simulink library "Chip_Library"  (R2018b)
settings: Solver=VariableStepAuto  StartTime=0.0  StopTime=10.0  RelTol=1e-3
settings Model: Creator=jon  LastModifiedBy=jon
settings DebuggingCC: LibraryContextMissingDiagnostic=none
settings SFSimCC: SimUseLocalCustomCode=off
settings RTWCC: RTWUseLocalCustomCode=off

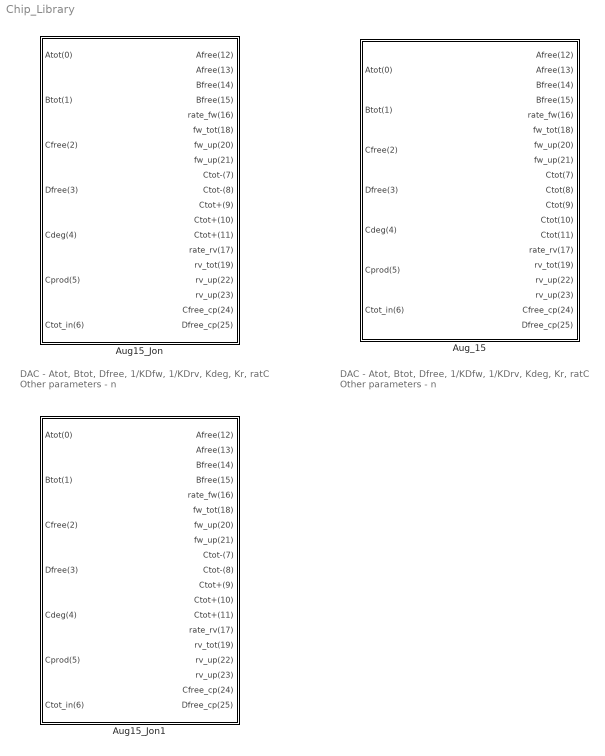
== system Chip_Library ==
  note: DAC - Atot, Btot, Dfree, 1/KDfw, 1/KDrv, Kdeg, Kr, ratC
      | Other parameters - n
  note: DAC - Atot, Btot, Dfree, 1/KDfw, 1/KDrv, Kdeg, Kr, ratC
      | Other parameters - n
  Aug15_Jon : Subsystem  mask{KDfw=1, KDrv=1, kr=1, kdeg=1, ratC=1, n=1, c_ic=0.01, A_FB_EN=0, B_FB_EN=0, FF_EN1=0, FF_EN2=0, FF_EN3=0, FF_EN4=0, Ctot_sw=0}
      mask prompts: KDfw "KD of forward reaction (KDfw)"; KDrv "KD of reverse reaction* (KDrv)"; kr "Reverse reaction rate (kr)"; kdeg "Degradation rate overall (kdeg)"; ratC "Degradation rate of C (ratC)"; n "Hill coefficient (n)"; c_ic "Initial condition of C (c_ic)"; A_FB_EN "Switch for Afree = Atot - ||| Ctot ||| (A_FB_EN)"; B_FB_EN "Switch for Bfree = Btot - ||| Ctot |||  (B_FB_EN)"; FF_EN1 "Switch for fw_up = C_prod - ||| rate_fw ||| (FF_EN1)"; FF_EN2 "Switch for fw_tot = C_prod + ||| rate_fw ||| (FF_EN2)"; FF_EN3 "Switch for rv_tot = C_deg+deg + ||| rate_rv ||| (FF_EN3)"; FF_EN4 "Switch for rv_up = C_deg+deg - ||| rate_rv ||| (FF_EN4)"; Ctot_sw "Switch for Ctot_in"
  Aug15_Jon1 : Subsystem  mask{Atot_cnst=0, Btot_cnst=0, Dfree_cnst=0, KDfw=1, KDrv=1, kr=1, kdeg=1, ratC=1, n=1, c_ic=0.01, A_FB_EN=0, B_FB_EN=0, sel_rate=1, sel_Ctot=1}
      mask prompts: Atot_cnst "Atot constant"; Btot_cnst "Btot constant"; Dfree_cnst "Dfree constant"; KDfw "KD of forward reaction (KDfw)"; KDrv "KD of reverse reaction* (KDrv)"; kr "Reverse reaction rate (kr)"; kdeg "Degradation rate overall (kdeg)"; ratC "Degradation rate of C (ratC)"; n "Hill coefficient (n)"; c_ic "Initial condition of C (c_ic)"; A_FB_EN "Switch for Afree = Atot - ||| Ctot ||| (A_FB_EN)"; B_FB_EN "Switch for Bfree = Btot - ||| Ctot |||  (B_FB_EN)"; sel_rate "fw_up, fw_tot, rv_tot, rv_up (Default=1: off on on off)"; sel_Ctot "Switch for Ctot_in (Default=1 : off)"
  Aug_15 : Subsystem  mask{KDfw=1, kr=1, kdeg=1, ratC=1, KDrv=1, n=1}

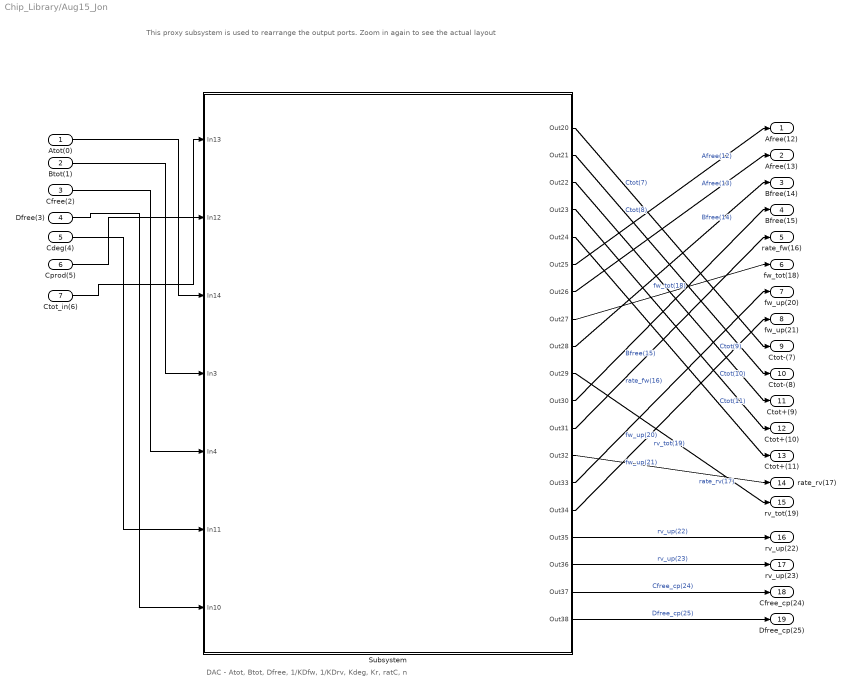
== system Chip_Library/Aug15_Jon ==
  note: This proxy subsystem is used to rearrange the output ports.
      | Zoom in again to see the actual layout
  note: DAC - Atot, Btot, Dfree, 1/KDfw, 1/KDrv, Kdeg, Kr, ratC, n
  Atot(0) : Inport
  Btot(1) : Inport  Port=2
  Cfree(2) : Inport  Port=3
  Dfree(3) : Inport  Port=4
  Cdeg(4) : Inport  Port=5
  Cprod(5) : Inport  Port=6
  Ctot_in(6) : Inport  Port=7
  Subsystem : Subsystem
  Afree(12) : Outport
  Afree(13) : Outport  Port=2
  Bfree(14) : Outport  Port=3
  Bfree(15) : Outport  Port=4
  rate_fw(16) : Outport  Port=5
  fw_tot(18) : Outport  Port=6
  fw_up(20) : Outport  Port=7
  fw_up(21) : Outport  Port=8
  Ctot-(7) : Outport  Port=9
  Ctot-(8) : Outport  Port=10
  Ctot+(9) : Outport  Port=11
  Ctot+(10) : Outport  Port=12
  Ctot+(11) : Outport  Port=13
  rate_rv(17) : Outport  Port=14
  rv_tot(19) : Outport  Port=15
  rv_up(22) : Outport  Port=16
  rv_up(23) : Outport  Port=17
  Cfree_cp(24) : Outport  Port=18
  Dfree_cp(25) : Outport  Port=19
  wires:
  Subsystem/8(Out27) -> fw_tot(18)/1  "fw_tot(18)"
  Subsystem/16(Out35) -> rv_up(22)/1  "rv_up(22)"
  Subsystem/3(Out22) -> Ctot+(9)/1  "Ctot(9)"
  Ctot_in(6)/1 -> Subsystem/1(In13)
  Cdeg(4)/1 -> Subsystem/6(In11)
  Cfree(2)/1 -> Subsystem/5(In4)
  Subsystem/9(Out28) -> Bfree(14)/1  "Bfree(14)"
  Atot(0)/1 -> Subsystem/3(In14)
  Subsystem/1(Out20) -> Ctot-(7)/1  "Ctot(7)"
  Btot(1)/1 -> Subsystem/4(In3)
  Subsystem/2(Out21) -> Ctot-(8)/1  "Ctot(8)"
  Subsystem/11(Out30) -> Bfree(15)/1  "Bfree(15)"
  Subsystem/18(Out37) -> Cfree_cp(24)/1  "Cfree_cp(24)"
  Subsystem/5(Out24) -> Ctot+(11)/1  "Ctot(11)"
  Dfree(3)/1 -> Subsystem/7(In10)
  Cprod(5)/1 -> Subsystem/2(In12)
  Subsystem/15(Out34) -> fw_up(21)/1  "fw_up(21)"
  Subsystem/4(Out23) -> Ctot+(10)/1  "Ctot(10)"
  Subsystem/19(Out38) -> Dfree_cp(25)/1  "Dfree_cp(25)"
  Subsystem/14(Out33) -> fw_up(20)/1  "fw_up(20)"
  Subsystem/6(Out25) -> Afree(12)/1  "Afree(12)"
  Subsystem/12(Out31) -> rate_fw(16)/1  "rate_fw(16)"
  Subsystem/7(Out26) -> Afree(13)/1  "Afree(13)"
  Subsystem/13(Out32) -> rate_rv(17)/1  "rate_rv(17)"
  Subsystem/17(Out36) -> rv_up(23)/1  "rv_up(23)"
  Subsystem/10(Out29) -> rv_tot(19)/1  "rv_tot(19)"

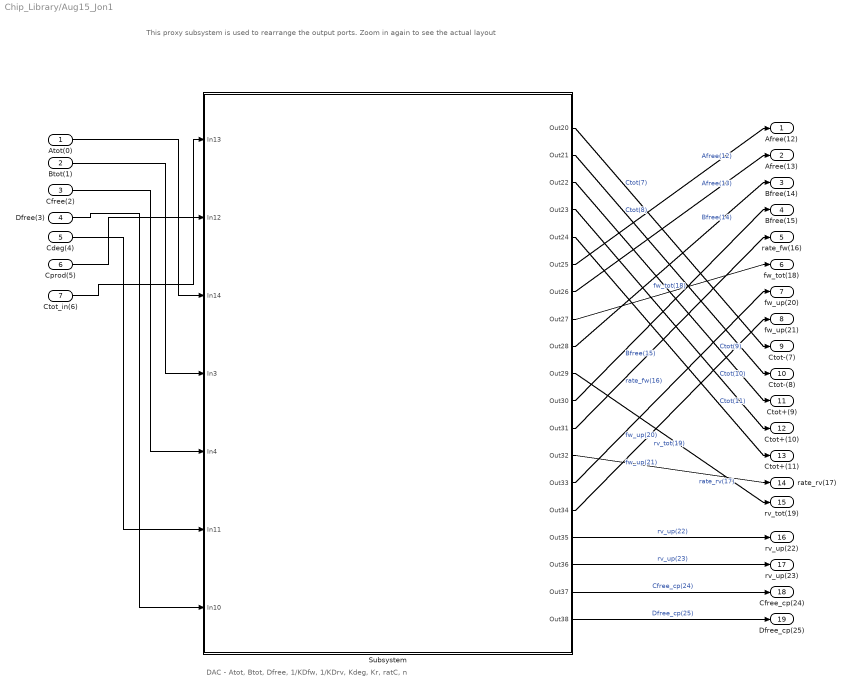
== system Chip_Library/Aug15_Jon1 ==
  note: This proxy subsystem is used to rearrange the output ports.
      | Zoom in again to see the actual layout
  note: DAC - Atot, Btot, Dfree, 1/KDfw, 1/KDrv, Kdeg, Kr, ratC, n
  Atot(0) : Inport
  Btot(1) : Inport  Port=2
  Cfree(2) : Inport  Port=3
  Dfree(3) : Inport  Port=4
  Cdeg(4) : Inport  Port=5
  Cprod(5) : Inport  Port=6
  Ctot_in(6) : Inport  Port=7
  Subsystem : Subsystem
  Afree(12) : Outport
  Afree(13) : Outport  Port=2
  Bfree(14) : Outport  Port=3
  Bfree(15) : Outport  Port=4
  rate_fw(16) : Outport  Port=5
  fw_tot(18) : Outport  Port=6
  fw_up(20) : Outport  Port=7
  fw_up(21) : Outport  Port=8
  Ctot-(7) : Outport  Port=9
  Ctot-(8) : Outport  Port=10
  Ctot+(9) : Outport  Port=11
  Ctot+(10) : Outport  Port=12
  Ctot+(11) : Outport  Port=13
  rate_rv(17) : Outport  Port=14
  rv_tot(19) : Outport  Port=15
  rv_up(22) : Outport  Port=16
  rv_up(23) : Outport  Port=17
  Cfree_cp(24) : Outport  Port=18
  Dfree_cp(25) : Outport  Port=19
  wires:
  Subsystem/8(Out27) -> fw_tot(18)/1  "fw_tot(18)"
  Subsystem/16(Out35) -> rv_up(22)/1  "rv_up(22)"
  Subsystem/3(Out22) -> Ctot+(9)/1  "Ctot(9)"
  Ctot_in(6)/1 -> Subsystem/1(In13)
  Cdeg(4)/1 -> Subsystem/6(In11)
  Cfree(2)/1 -> Subsystem/5(In4)
  Subsystem/9(Out28) -> Bfree(14)/1  "Bfree(14)"
  Atot(0)/1 -> Subsystem/3(In14)
  Subsystem/1(Out20) -> Ctot-(7)/1  "Ctot(7)"
  Btot(1)/1 -> Subsystem/4(In3)
  Subsystem/2(Out21) -> Ctot-(8)/1  "Ctot(8)"
  Subsystem/11(Out30) -> Bfree(15)/1  "Bfree(15)"
  Subsystem/18(Out37) -> Cfree_cp(24)/1  "Cfree_cp(24)"
  Subsystem/5(Out24) -> Ctot+(11)/1  "Ctot(11)"
  Dfree(3)/1 -> Subsystem/7(In10)
  Cprod(5)/1 -> Subsystem/2(In12)
  Subsystem/15(Out34) -> fw_up(21)/1  "fw_up(21)"
  Subsystem/4(Out23) -> Ctot+(10)/1  "Ctot(10)"
  Subsystem/19(Out38) -> Dfree_cp(25)/1  "Dfree_cp(25)"
  Subsystem/14(Out33) -> fw_up(20)/1  "fw_up(20)"
  Subsystem/6(Out25) -> Afree(12)/1  "Afree(12)"
  Subsystem/12(Out31) -> rate_fw(16)/1  "rate_fw(16)"
  Subsystem/7(Out26) -> Afree(13)/1  "Afree(13)"
  Subsystem/13(Out32) -> rate_rv(17)/1  "rate_rv(17)"
  Subsystem/17(Out36) -> rv_up(23)/1  "rv_up(23)"
  Subsystem/10(Out29) -> rv_tot(19)/1  "rv_tot(19)"

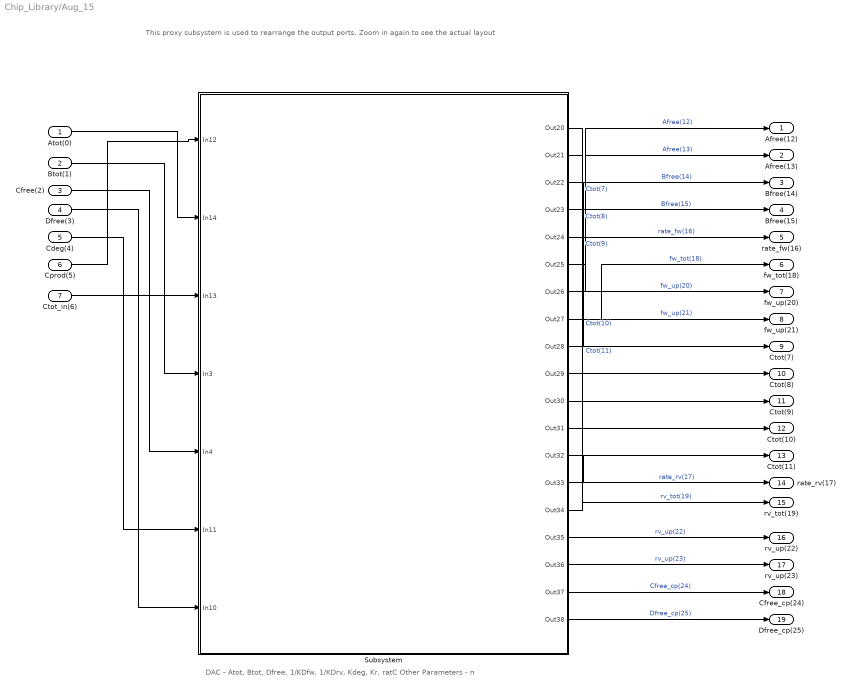
== system Chip_Library/Aug_15 ==
  note: This proxy subsystem is used to rearrange the output ports.
      | Zoom in again to see the actual layout
  note: DAC - Atot, Btot, Dfree, 1/KDfw, 1/KDrv, Kdeg, Kr, ratC
      | Other Parameters - n
  Atot(0) : Inport
  Btot(1) : Inport  Port=2
  Cfree(2) : Inport  Port=3
  Dfree(3) : Inport  Port=4
  Cdeg(4) : Inport  Port=5
  Cprod(5) : Inport  Port=6
  Ctot_in(6) : Inport  Port=7
  Subsystem : Subsystem
  Afree(12) : Outport
  Afree(13) : Outport  Port=2
  Bfree(14) : Outport  Port=3
  Bfree(15) : Outport  Port=4
  rate_fw(16) : Outport  Port=5
  fw_tot(18) : Outport  Port=6
  fw_up(20) : Outport  Port=7
  fw_up(21) : Outport  Port=8
  Ctot(7) : Outport  Port=9
  Ctot(8) : Outport  Port=10
  Ctot(9) : Outport  Port=11
  Ctot(10) : Outport  Port=12
  Ctot(11) : Outport  Port=13
  rate_rv(17) : Outport  Port=14
  rv_tot(19) : Outport  Port=15
  rv_up(22) : Outport  Port=16
  rv_up(23) : Outport  Port=17
  Cfree_cp(24) : Outport  Port=18
  Dfree_cp(25) : Outport  Port=19
  wires:
  Subsystem/8(Out27) -> fw_tot(18)/1  "fw_tot(18)"
  Subsystem/16(Out35) -> rv_up(22)/1  "rv_up(22)"
  Subsystem/3(Out22) -> Ctot(9)/1  "Ctot(9)"
  Ctot_in(6)/1 -> Subsystem/3(In13)
  Cdeg(4)/1 -> Subsystem/6(In11)
  Cfree(2)/1 -> Subsystem/5(In4)
  Subsystem/9(Out28) -> Bfree(14)/1  "Bfree(14)"
  Atot(0)/1 -> Subsystem/2(In14)
  Subsystem/1(Out20) -> Ctot(7)/1  "Ctot(7)"
  Btot(1)/1 -> Subsystem/4(In3)
  Subsystem/2(Out21) -> Ctot(8)/1  "Ctot(8)"
  Subsystem/11(Out30) -> Bfree(15)/1  "Bfree(15)"
  Subsystem/18(Out37) -> Cfree_cp(24)/1  "Cfree_cp(24)"
  Subsystem/5(Out24) -> Ctot(11)/1  "Ctot(11)"
  Dfree(3)/1 -> Subsystem/7(In10)
  Cprod(5)/1 -> Subsystem/1(In12)
  Subsystem/15(Out34) -> fw_up(21)/1  "fw_up(21)"
  Subsystem/4(Out23) -> Ctot(10)/1  "Ctot(10)"
  Subsystem/19(Out38) -> Dfree_cp(25)/1  "Dfree_cp(25)"
  Subsystem/14(Out33) -> fw_up(20)/1  "fw_up(20)"
  Subsystem/6(Out25) -> Afree(12)/1  "Afree(12)"
  Subsystem/12(Out31) -> rate_fw(16)/1  "rate_fw(16)"
  Subsystem/7(Out26) -> Afree(13)/1  "Afree(13)"
  Subsystem/13(Out32) -> rate_rv(17)/1  "rate_rv(17)"
  Subsystem/17(Out36) -> rv_up(23)/1  "rv_up(23)"
  Subsystem/10(Out29) -> rv_tot(19)/1  "rv_tot(19)"

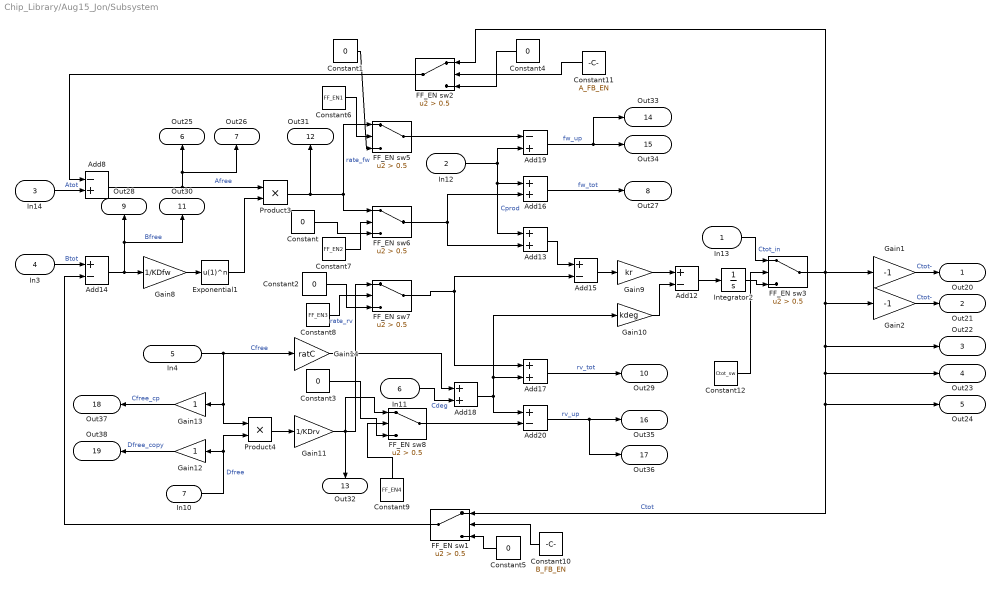
== system Chip_Library/Aug15_Jon/Subsystem ==
  In13 : Inport
  In12 : Inport  Port=2
  In14 : Inport  Port=3
  In3 : Inport  Port=4
  In4 : Inport  Port=5
  In11 : Inport  Port=6
  In10 : Inport  Port=7
  Add{12,14..15,20} (4 alike) : Sum  Inputs=+-
  Add{13,16..18} (4 alike) : Sum
  Add19 : Sum  Inputs=-+
  Add8 : Sum  Inputs=-+
  Constant{,1..5} (6 alike) : Constant  Value=0
  Constant10 : Constant  Value=B_FB_EN
  Constant11 : Constant  Value=A_FB_EN
  Constant12 : Constant  Value=Ctot_sw
  Constant6 : Constant  Value=FF_EN1
  Constant7 : Constant  Value=FF_EN2
  Constant8 : Constant  Value=FF_EN3
  Constant9 : Constant  Value=FF_EN4
  Exponential1 : Fcn  Expr=u(1)^n
  FF_EN sw{1..3,5..8} (7 alike) : Switch  Criteria=u2 > Threshold  Threshold=0.5
  Gain1 : Gain  Gain=-1
  Gain10 : Gain  Gain=kdeg
  Gain11 : Gain  Gain=1/KDrv
  Gain12 : Gain
  Gain13 : Gain
  Gain14 : Gain  Gain=ratC
  Gain2 : Gain  Gain=-1
  Gain8 : Gain  Gain=1/KDfw
  Gain9 : Gain  Gain=kr
  Integrator2 : Integrator  InitialCondition=c_ic
  Product3 : Product  RndMeth=Zero
  Product4 : Product  RndMeth=Zero
  Out20 : Outport
  Out21 : Outport  Port=2
  Out22 : Outport  Port=3
  Out23 : Outport  Port=4
  Out24 : Outport  Port=5
  Out25 : Outport  Port=6
  Out26 : Outport  Port=7
  Out27 : Outport  Port=8
  Out28 : Outport  Port=9
  Out29 : Outport  Port=10
  Out30 : Outport  Port=11
  Out31 : Outport  Port=12
  Out32 : Outport  Port=13
  Out33 : Outport  Port=14
  Out34 : Outport  Port=15
  Out35 : Outport  Port=16
  Out36 : Outport  Port=17
  Out37 : Outport  Port=18
  Out38 : Outport  Port=19
  wires:
  Constant5/1 -> FF_EN sw1/3
  Constant3/1 -> FF_EN sw8/3
  Gain10/1 -> Add12/2
  Add15/1 -> Gain9/1
  Integrator2/1 -> FF_EN sw3/3
  Gain14/1 -> Add18/1
  In14/1 -> Add8/2  "Atot"
  Add13/1 -> Add15/1
  Add18/1 -> Add20/1, Gain10/1, Add17/2
  In10/1 -> Gain12/1, Product4/2  "Dfree"
  Product4/1 -> Gain11/1
  Add19/1 -> Out34/1, Out33/1  "fw_up"
  Constant1/1 -> FF_EN sw5/3
  Add8/1 -> Product3/1, Out26/1, Out25/1  "Afree"
  FF_EN sw1/1 -> Add14/2
  Constant2/1 -> FF_EN sw7/3
  Add20/1 -> Out36/1, Out35/1  "rv_up"
  FF_EN sw3/1 -> Gain1/1, FF_EN sw2/1, Gain2/1, FF_EN sw1/1, Out24/1, Out23/1, Out22/1  "Ctot"
  In13/1 -> FF_EN sw3/1  "Ctot_in"
  Gain11/1 -> Out32/1, FF_EN sw8/1, FF_EN sw7/1  "rate_rv"
  Gain9/1 -> Add12/1
  In12/1 -> Add19/2, Add16/1, Add13/1  "Cprod"
  Add12/1 -> Integrator2/1
  Add16/1 -> Out27/1  "fw_tot"
  Constant4/1 -> FF_EN sw2/3
  Exponential1/1 -> Product3/2
  FF_EN sw6/1 -> Add16/2, Add13/2
  FF_EN sw2/1 -> Add8/1
  Gain13/1 -> Out37/1  "Cfree_cp"
  In11/1 -> Add18/2  "Cdeg"
  Add14/1 -> Out30/1, Out28/1, Gain8/1  "Bfree"
  FF_EN sw8/1 -> Add20/2
  In4/1 -> Gain14/1, Product4/1, Gain13/1  "Cfree"
  Gain8/1 -> Exponential1/1
  Gain12/1 -> Out38/1  "Dfree_copy"
  Constant/1 -> FF_EN sw6/3
  Product3/1 -> Out31/1, FF_EN sw6/1, FF_EN sw5/1  "rate_fw"
  Add17/1 -> Out29/1  "rv_tot"
  FF_EN sw7/1 -> Add17/1, Add15/2
  FF_EN sw5/1 -> Add19/1
  In3/1 -> Add14/1  "Btot"
  Constant6/1 -> FF_EN sw5/2
  Constant7/1 -> FF_EN sw6/2
  Constant8/1 -> FF_EN sw7/2
  Constant9/1 -> FF_EN sw8/2
  Constant10/1 -> FF_EN sw1/2
  Constant11/1 -> FF_EN sw2/2
  Constant12/1 -> FF_EN sw3/2
  Gain1/1 -> Out20/1  "Ctot-"
  Gain2/1 -> Out21/1  "Ctot-"

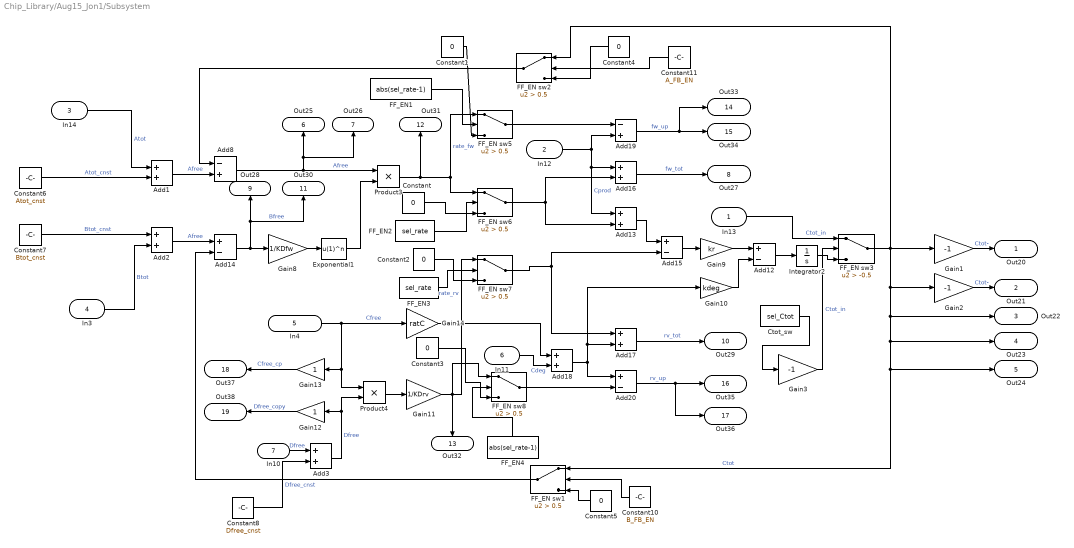
== system Chip_Library/Aug15_Jon1/Subsystem ==
  In13 : Inport
  In12 : Inport  Port=2
  In14 : Inport  Port=3
  In3 : Inport  Port=4
  In4 : Inport  Port=5
  In11 : Inport  Port=6
  In10 : Inport  Port=7
  Add{1..3,13,16..18} (7 alike) : Sum
  Add{12,14..15,20} (4 alike) : Sum  Inputs=+-
  Add19 : Sum  Inputs=-+
  Add8 : Sum  Inputs=-+
  Constant{,1..5} (6 alike) : Constant  Value=0
  Constant10 : Constant  Value=B_FB_EN
  Constant11 : Constant  Value=A_FB_EN
  Constant6 : Constant  Value=Atot_cnst
  Constant7 : Constant  Value=Btot_cnst
  Constant8 : Constant  Value=Dfree_cnst
  Ctot_sw : Constant  Value=sel_Ctot
  Exponential1 : Fcn  Expr=u(1)^n
  FF_EN sw{1..2,5..8} (6 alike) : Switch  Criteria=u2 > Threshold  Threshold=0.5
  FF_EN sw3 : Switch  Criteria=u2 > Threshold  Threshold=-0.5
  FF_EN1 : Constant  Value=abs(sel_rate-1)
  FF_EN2 : Constant  Value=sel_rate
  FF_EN3 : Constant  Value=sel_rate
  FF_EN4 : Constant  Value=abs(sel_rate-1)
  Gain1 : Gain  Gain=-1
  Gain10 : Gain  Gain=kdeg
  Gain11 : Gain  Gain=1/KDrv
  Gain12 : Gain
  Gain13 : Gain
  Gain14 : Gain  Gain=ratC
  Gain2 : Gain  Gain=-1
  Gain3 : Gain  Gain=-1
  Gain8 : Gain  Gain=1/KDfw
  Gain9 : Gain  Gain=kr
  Integrator2 : Integrator  InitialCondition=c_ic
  Product3 : Product  RndMeth=Zero
  Product4 : Product  RndMeth=Zero
  Out20 : Outport
  Out21 : Outport  Port=2
  Out22 : Outport  Port=3
  Out23 : Outport  Port=4
  Out24 : Outport  Port=5
  Out25 : Outport  Port=6
  Out26 : Outport  Port=7
  Out27 : Outport  Port=8
  Out28 : Outport  Port=9
  Out29 : Outport  Port=10
  Out30 : Outport  Port=11
  Out31 : Outport  Port=12
  Out32 : Outport  Port=13
  Out33 : Outport  Port=14
  Out34 : Outport  Port=15
  Out35 : Outport  Port=16
  Out36 : Outport  Port=17
  Out37 : Outport  Port=18
  Out38 : Outport  Port=19
  wires:
  Constant5/1 -> FF_EN sw1/3
  Constant3/1 -> FF_EN sw8/3
  Gain10/1 -> Add12/2
  Add15/1 -> Gain9/1
  Integrator2/1 -> FF_EN sw3/3
  Gain14/1 -> Add18/1
  In14/1 -> Add1/1  "Atot"
  Add13/1 -> Add15/1
  Add18/1 -> Add20/1, Gain10/1, Add17/2
  Add3/1 -> Gain12/1, Product4/2  "Dfree"
  Product4/1 -> Gain11/1
  Add19/1 -> Out34/1, Out33/1  "fw_up"
  Constant1/1 -> FF_EN sw5/3
  Add8/1 -> Product3/1, Out26/1, Out25/1  "Afree"
  FF_EN sw1/1 -> Add14/2
  Constant2/1 -> FF_EN sw7/3
  Add20/1 -> Out36/1, Out35/1  "rv_up"
  FF_EN sw3/1 -> Gain1/1, FF_EN sw2/1, Gain2/1, FF_EN sw1/1, Out24/1, Out23/1, Out22/1  "Ctot"
  In13/1 -> FF_EN sw3/1  "Ctot_in"
  Gain11/1 -> Out32/1, FF_EN sw8/1, FF_EN sw7/1  "rate_rv"
  Gain9/1 -> Add12/1
  In12/1 -> Add19/2, Add16/1, Add13/1  "Cprod"
  Add12/1 -> Integrator2/1
  Add16/1 -> Out27/1  "fw_tot"
  Constant4/1 -> FF_EN sw2/3
  Exponential1/1 -> Product3/2
  FF_EN sw6/1 -> Add16/2, Add13/2
  FF_EN sw2/1 -> Add8/1
  Gain13/1 -> Out37/1  "Cfree_cp"
  In11/1 -> Add18/2  "Cdeg"
  Add14/1 -> Out30/1, Out28/1, Gain8/1  "Bfree"
  FF_EN sw8/1 -> Add20/2
  In4/1 -> Gain14/1, Product4/1, Gain13/1  "Cfree"
  Gain8/1 -> Exponential1/1
  Gain12/1 -> Out38/1  "Dfree_copy"
  Constant/1 -> FF_EN sw6/3
  Product3/1 -> Out31/1, FF_EN sw6/1, FF_EN sw5/1  "rate_fw"
  Add17/1 -> Out29/1  "rv_tot"
  FF_EN sw7/1 -> Add17/1, Add15/2
  FF_EN sw5/1 -> Add19/1
  FF_EN1/1 -> FF_EN sw5/2
  FF_EN2/1 -> FF_EN sw6/2
  FF_EN3/1 -> FF_EN sw7/2
  FF_EN4/1 -> FF_EN sw8/2
  Constant10/1 -> FF_EN sw1/2
  Constant11/1 -> FF_EN sw2/2
  Ctot_sw/1 -> Gain3/1
  Gain1/1 -> Out20/1  "Ctot-"
  Gain2/1 -> Out21/1  "Ctot-"
  Gain3/1 -> FF_EN sw3/2  "Ctot_in"
  Add1/1 -> Add8/2  "Afree"
  In3/1 -> Add2/2  "Btot"
  Add2/1 -> Add14/1  "Afree"
  Constant6/1 -> Add1/2  "Atot_cnst"
  Constant7/1 -> Add2/1  "Btot_cnst"
  In10/1 -> Add3/1  "Dfree"
  Constant8/1 -> Add3/2  "Dfree_cnst"

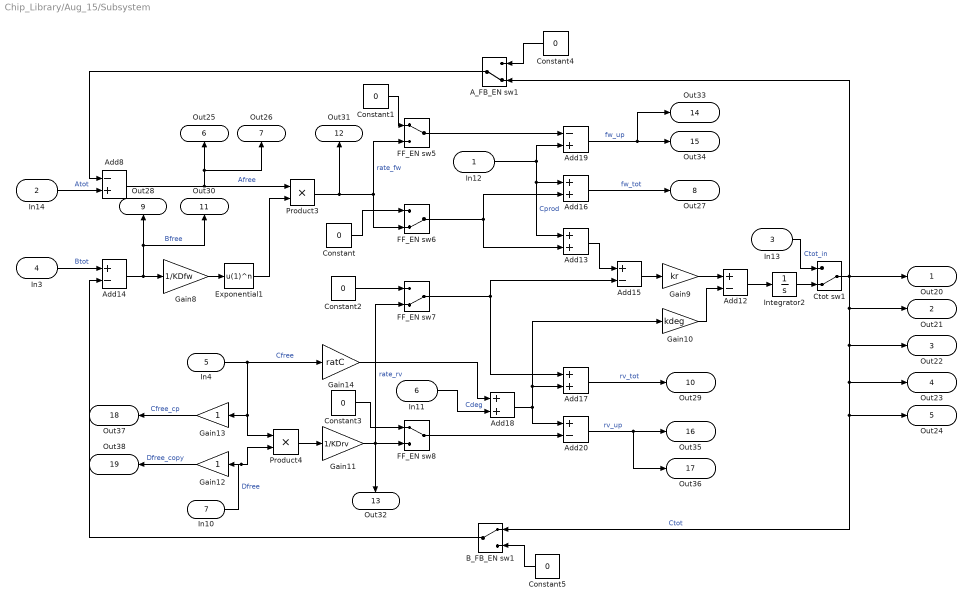
== system Chip_Library/Aug_15/Subsystem ==
  In12 : Inport
  In14 : Inport  Port=2
  In13 : Inport  Port=3
  In3 : Inport  Port=4
  In4 : Inport  Port=5
  In11 : Inport  Port=6
  In10 : Inport  Port=7
  A_FB_EN sw1 : ManualSwitch  CurrentSetting=0
  Add{12,14..15,20} (4 alike) : Sum  Inputs=+-
  Add{13,16..18} (4 alike) : Sum
  Add19 : Sum  Inputs=-+
  Add8 : Sum  Inputs=-+
  B_FB_EN sw1 : ManualSwitch
  Constant{,1..5} (6 alike) : Constant  Value=0
  Ctot sw1 : ManualSwitch  CurrentSetting=0
  Exponential1 : Fcn  Expr=u(1)^n
  FF_EN sw5 : ManualSwitch
  FF_EN sw6 : ManualSwitch  CurrentSetting=0
  FF_EN sw7 : ManualSwitch  CurrentSetting=0
  FF_EN sw8 : ManualSwitch
  Gain10 : Gain  Gain=kdeg
  Gain11 : Gain  Gain=1/KDrv
  Gain12 : Gain
  Gain13 : Gain
  Gain14 : Gain  Gain=ratC
  Gain8 : Gain  Gain=1/KDfw
  Gain9 : Gain  Gain=kr
  Integrator2 : Integrator  InitialCondition=100
  Product3 : Product  RndMeth=Zero
  Product4 : Product  RndMeth=Zero
  Out20 : Outport
  Out21 : Outport  Port=2
  Out22 : Outport  Port=3
  Out23 : Outport  Port=4
  Out24 : Outport  Port=5
  Out25 : Outport  Port=6
  Out26 : Outport  Port=7
  Out27 : Outport  Port=8
  Out28 : Outport  Port=9
  Out29 : Outport  Port=10
  Out30 : Outport  Port=11
  Out31 : Outport  Port=12
  Out32 : Outport  Port=13
  Out33 : Outport  Port=14
  Out34 : Outport  Port=15
  Out35 : Outport  Port=16
  Out36 : Outport  Port=17
  Out37 : Outport  Port=18
  Out38 : Outport  Port=19
  wires:
  Constant5/1 -> B_FB_EN sw1/2
  Constant3/1 -> FF_EN sw8/1
  Gain10/1 -> Add12/2
  Add15/1 -> Gain9/1
  Integrator2/1 -> Ctot sw1/2
  Gain14/1 -> Add18/1
  In14/1 -> Add8/2  "Atot"
  Add13/1 -> Add15/1
  Add18/1 -> Add20/1, Gain10/1, Add17/2
  In10/1 -> Product4/2, Gain12/1  "Dfree"
  Product4/1 -> Gain11/1
  Add19/1 -> Out34/1, Out33/1  "fw_up"
  Constant1/1 -> FF_EN sw5/1
  Add8/1 -> Product3/1, Out26/1, Out25/1  "Afree"
  B_FB_EN sw1/1 -> Add14/2
  Constant2/1 -> FF_EN sw7/1
  Add20/1 -> Out36/1, Out35/1  "rv_up"
  Ctot sw1/1 -> Out20/1, A_FB_EN sw1/2, Out21/1, Out22/1, Out23/1, Out24/1, B_FB_EN sw1/1  "Ctot"
  In13/1 -> Ctot sw1/1  "Ctot_in"
  Gain11/1 -> Out32/1, FF_EN sw7/2, FF_EN sw8/2  "rate_rv"
  Gain9/1 -> Add12/1
  In12/1 -> Add19/2, Add16/1, Add13/1  "Cprod"
  Add12/1 -> Integrator2/1
  Add16/1 -> Out27/1  "fw_tot"
  Constant4/1 -> A_FB_EN sw1/1
  Exponential1/1 -> Product3/2
  FF_EN sw6/1 -> Add16/2, Add13/2
  A_FB_EN sw1/1 -> Add8/1
  Gain13/1 -> Out37/1  "Cfree_cp"
  In11/1 -> Add18/2  "Cdeg"
  Add14/1 -> Out30/1, Out28/1, Gain8/1  "Bfree"
  FF_EN sw8/1 -> Add20/2
  In4/1 -> Gain14/1, Product4/1, Gain13/1  "Cfree"
  Gain8/1 -> Exponential1/1
  Gain12/1 -> Out38/1  "Dfree_copy"
  Constant/1 -> FF_EN sw6/1
  Product3/1 -> Out31/1, FF_EN sw6/2, FF_EN sw5/2  "rate_fw"
  Add17/1 -> Out29/1  "rv_tot"
  FF_EN sw7/1 -> Add17/1, Add15/2
  FF_EN sw5/1 -> Add19/1
  In3/1 -> Add14/1  "Btot"
